simulink model "example_Radiation_Division"  (R2018b)
settings: Solver=ode45  StartTime=0.0  StopTime=365*24*3600  MaxStep=100  RelTol=1e-3  EnableMultiTasking=on
undefined symbols (not defined in the file): path_carnot
libraries: carnot x2
settings Model: Creator=drhf  LastModifiedBy=drhf
settings DataIOCC: LimitDataPoints=on  SaveFormat=Array  SignalLoggingSaveFormat=ModelDataLogs
settings OptimizationCC: ExpressionDepthLimit=2147483647  LifeSpan=inf
settings DebuggingCC: UnderspecifiedInitializationDetection=Classic  MergeDetectMultiDrivingBlocksExec=none  SolverPrmCheckMsg=warning  FcnCallInpInsideContextMsg=warning  StateNameClashWarn=warning  SFUnexpectedBacktrackingDiag=warning  SFNoUnconditionalDefaultTransitionDiag=warning  SFExecutionAtInitializationDiag=none
settings HardwareCC: ProdBitPerPointer=32  ProdBitPerSizeT=32  ProdBitPerPtrDiffT=32  ProdLargestAtomicFloat=None  ProdIntDivRoundTo=Undefined  ProdEndianess=Unspecified  ProdWordSize=32  ProdHWDeviceType=32-bit Generic
settings ModelReferenceCC: PropagateSignalLabelsOutOfModel=off
settings SFSimCC: SimUseLocalCustomCode=off
settings RTWCC: RTWUseLocalCustomCode=off
settings CodeAppCC: StateflowObjectComments=on
settings GRTTargetCC: TargetLangStandard=C89/C90 (ANSI)  GeneratePreprocessorConditionals=Disable all  CombineOutputUpdateFcns=off  GRTInterface=on
settings ConfigComp: CovMetricSettings=dw  CovHtmlReporting=on  CovSaveCumulativeToWorkspaceVar=on  CovSaveSingleToWorkspaceVar=on  CovExternalEMLEnable=off

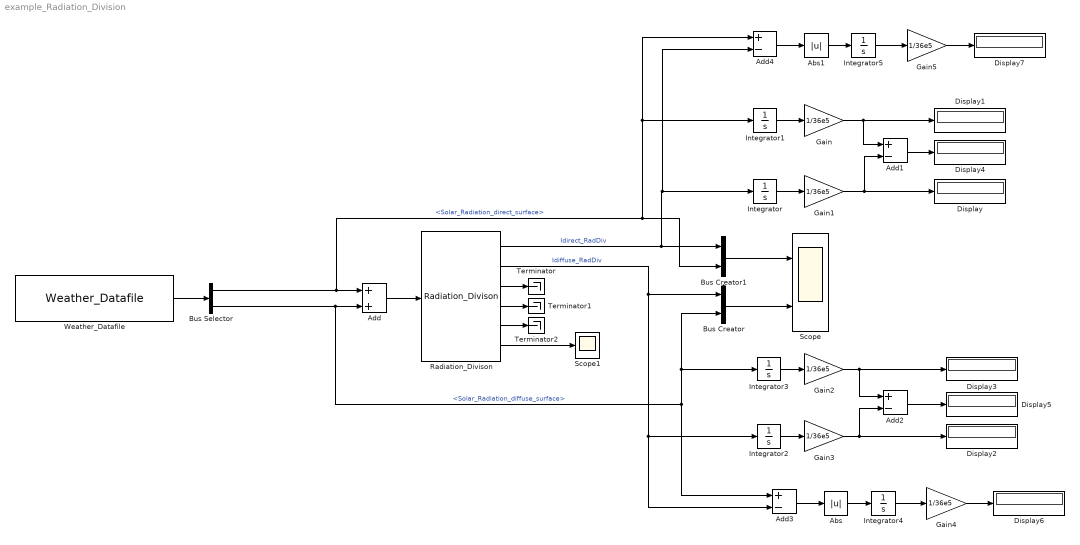
== system example_Radiation_Division ==
  Abs : Abs
  Abs1 : Abs
  Add : Sum
  Add{1..4} (4 alike) : Sum  Inputs=+-
  Bus Creator : BusCreator  Inputs=2
  Bus Creator1 : BusCreator  Inputs=2
  Bus Selector : BusSelector  OutputSignals=Solar_Radiation_direct_surface,Solar_Radiation_diffuse_surface
  Display{,1..7} (8 alike) : Display
  Gain{,1..5} (6 alike) : Gain  Gain=1/36e5
  Integrator{,1..5} (6 alike) : Integrator
  Radiation_Divison : carnot/Basic/Weather_and_Sun/Radiation_Divison  latitude=52.393800 % TRY 2016 Potsdam / Germany  longitude=-13.065100 % TRY 2016 Potsdam / Germany  longitude0="-15  % CET"
      settings: SourceProductName=Carnot
  Scope : Scope  NumInputPorts=2
  Scope1 : Scope
  Terminator : Terminator
  Terminator1 : Terminator
  Terminator2 : Terminator
  Weather_Datafile : carnot/Weather/Weather_Datafile  PathName=path_carnot('data')  FileName='DE_TRY2016_Potsdam_averageYear.mat'  UserParam=off  VariableName=DE_TRY2010_04_averageYear  SampleTime=3600
      settings: SourceProductName=Carnot
  wires:
  Radiation_Divison/1 -> Add4/2, Integrator/1, Bus Creator1/1  "Idirect_RadDiv"
  Radiation_Divison/2 -> Add3/2, Integrator2/1, Bus Creator/1  "Idiffuse_RadDiv"
  Radiation_Divison/3 -> Terminator/1
  Radiation_Divison/4 -> Terminator1/1
  Radiation_Divison/5 -> Terminator2/1
  Bus Selector/1 -> Add/1, Add4/1, Integrator1/1, Bus Creator1/2  "<Solar_Radiation_direct_surface>"
  Weather_Datafile/1 -> Bus Selector/1
  Add/1 -> Radiation_Divison/1
  Bus Selector/2 -> Add/2, Integrator3/1, Bus Creator/2, Add3/1  "<Solar_Radiation_diffuse_surface>"
  Bus Creator1/1 -> Scope/1
  Bus Creator/1 -> Scope/2
  Integrator/1 -> Gain1/1
  Integrator1/1 -> Gain/1
  Integrator3/1 -> Gain2/1
  Integrator2/1 -> Gain3/1
  Gain/1 -> Add1/1, Display1/1
  Gain1/1 -> Add1/2, Display/1
  Gain2/1 -> Add2/1, Display3/1
  Gain3/1 -> Add2/2, Display2/1
  Add1/1 -> Display4/1
  Add2/1 -> Display5/1
  Gain4/1 -> Display6/1
  Integrator4/1 -> Gain4/1
  Add3/1 -> Abs/1
  Abs/1 -> Integrator4/1
  Abs1/1 -> Integrator5/1
  Add4/1 -> Abs1/1
  Integrator5/1 -> Gain5/1
  Gain5/1 -> Display7/1
  Radiation_Divison/6 -> Scope1/1
